simulink model "P1Q6"  (R2017a)
settings: Solver=VariableStepAuto  StartTime=0.0  StopTime=10.0  RelTol=1e-3
settings Model: Creator=ifaruk  LastModifiedBy=ifaruk

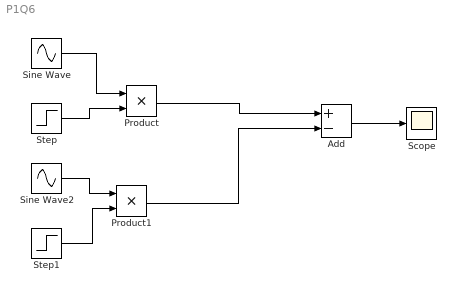
== system P1Q6 ==
  Add : Sum  Inputs=+-
  Product : Product
  Product1 : Product
  Scope : Scope
  Sine Wave : Sin  SineType=Sample based  Amplitude=0.5  Samples=1000  SampleTime=0.001
  Sine Wave2 : Sin  SineType=Sample based  Amplitude=0.5  Samples=1000  SampleTime=0.001
  Step : Step  Time=2  SampleTime=0
  Step1 : Step  Time=4  SampleTime=0
  wires:
  Sine Wave/1 -> Product/1
  Step/1 -> Product/2
  Sine Wave2/1 -> Product1/1
  Step1/1 -> Product1/2
  Product/1 -> Add/1
  Product1/1 -> Add/2
  Add/1 -> Scope/1
